simulink model "LABVALVSIMU2019a"  (R2019b)
settings: Solver=VariableStepAuto  StartTime=0.0  StopTime=50  RelTol=1e-3  EnableMultiTasking=on
libraries: simulink x1
settings Model: Creator=mateog  LastModifiedBy=gesro
settings DataIOCC: ReturnWorkspaceOutputs=off
settings OptimizationCC: LifeSpan=inf
settings DebuggingCC: SFUnexpectedBacktrackingDiag=warning  SFNoUnconditionalDefaultTransitionDiag=warning  ArithmeticOperatorsInVariantConditions=warning
settings SFSimCC: SimUseLocalCustomCode=off  CustomCodeUndefinedFunction=UseInterfaceOnly
settings RTWCC: RTWUseLocalCustomCode=off
settings CodeAppCC: StateflowObjectComments=on
settings GRTTargetCC: TargetLangStandard=C89/C90 (ANSI)
settings ConfigComp: CovMetricSettings=dw  CovHtmlReporting=on  CovSaveCumulativeToWorkspaceVar=on  CovSaveSingleToWorkspaceVar=on  CovExternalEMLEnable=off

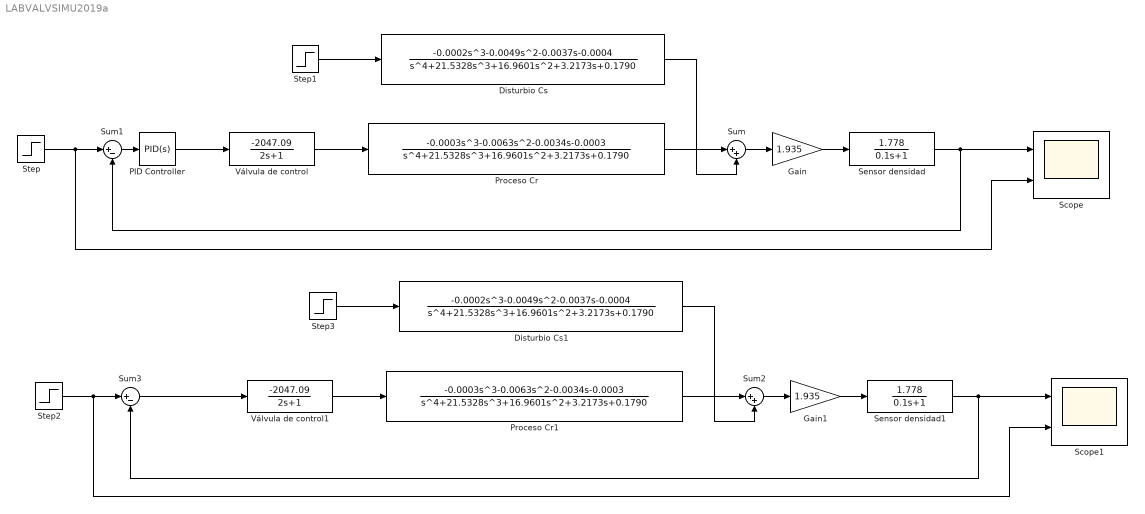
== system LABVALVSIMU2019a ==
  Disturbio Cs : TransferFcn  Numerator=[-0.0002 -0.0049 -0.0037 -0.0004]  Denominator=[1 21.5328 16.9601 3.2173 0.1790]
  Disturbio Cs1 : TransferFcn  Numerator=[-0.0002 -0.0049 -0.0037 -0.0004]  Denominator=[1 21.5328 16.9601 3.2173 0.1790]
  Gain : Gain  Gain=1.935
  Gain1 : Gain  Gain=1.935
  PID Controller : simulink/Continuous/PID Controller  Controller=PID  Form=Ideal  TimeDomain=Continuous-time  SampleTime=-1  IntegratorMethod=Forward Euler  FilterMethod=Forward Euler  ControllerParametersSource=internal  P=0.955917062218505  I=0.151469512178024  D=1.64233942236467  UseFilter=on  N=100  TunerSelectOption=Transfer Function Based (PID Tuner App)  InitialConditionSource=internal  InitialConditionForIntegrator=0  InitialConditionForFilter=0  DifferentiatorICPrevScaledInput=0  ExternalReset=none  TrackingMode=off  Kt=1  LimitOutput=off  UpperSaturationLimit=inf  LowerSaturationLimit=-inf  LinearizeAsGain=on  AntiWindupMode=none  Kb=1  POutMin=[]  POutMax=[]  IOutMin=[]  IOutMax=[]  DOutMin=[]  DOutMax=[]  NOutMin=[]  NOutMax=[]  SumOutMin=[]  SumOutMax=[]  SaturationOutMin=[]  SaturationOutMax=[]  PParamMin=[]  PParamMax=[]  IParamMin=[]  IParamMax=[]  DParamMin=[]  DParamMax=[]  NParamMin=[]  NParamMax=[]  KbParamMin=[]  KbParamMax=[]  KtParamMin=[]  KtParamMax=[]  KbOutMin=[]  KbOutMax=[]  KtOutMin=[]  KtOutMax=[]  IntegratorOutMin=[]  IntegratorOutMax=[]  FilterOutMin=[]  FilterOutMax=[]  SumI1OutMin=[]  SumI1OutMax=[]  SumI2OutMin=[]  SumI2OutMax=[]  SumI3OutMin=[]  SumI3OutMax=[]  SumI4OutMin=[]  SumI4OutMax=[]  SumDOutMin=[]  SumDOutMax=[]  DifferentiatorOutMin=[]  DifferentiatorOutMax=[]  FilterDiffOutCoefMin=[]  FilterDiffOutCoefMax=[]  ReciprocalOutMin=[]  ReciprocalOutMax=[]  SumDenOutMin=[]  SumDenOutMax=[]  SumNumOutMin=[]  SumNumOutMax=[]  DivideOutMin=[]  DivideOutMax=[]  IntegratorContinuousStateAttributes=''  IntegratorStateMustResolveToSignalObject=off  IntegratorRTWStateStorageClass=Auto  FilterContinuousStateAttributes=''  FilterStateMustResolveToSignalObject=off  FilterRTWStateStorageClass=Auto  ParallelPVariant=Passthrough  IdealPVariant=InternalParameters  IVariant=InternalParameters  DVariant=InternalParameters  IntegratorVariant=Continuous  SatVariant=Disabled  AWVariant=Passthrough  PCopyVariant=Disabled  TRVariant=Disabled  FdbkBlocksVariant=Forward  IdealPFdbkVariant=Disabled  SatFdbkVariant=Disabled  DerivativeFilterVariant=ContFilter  NVariant=InternalParameters  NCopyVariant=Disabled  FilterICVariant=InternalICsFilter  IntegratorICVariant=InternalICs  ExternalResetVariant=Disabled  TRSumVariant=Passthrough  SumFdbkVariant=Disabled  SumVariant=Sum_PID
  Proceso Cr : TransferFcn  Numerator=[-0.0003 -0.0063 -0.0034 -0.0003]  Denominator=[1 21.5328 16.9601 3.2173 0.1790]
  Proceso Cr1 : TransferFcn  Numerator=[-0.0003 -0.0063 -0.0034 -0.0003]  Denominator=[1 21.5328 16.9601 3.2173 0.1790]
  Scope : Scope  NumInputPorts=2
  Scope1 : Scope  NumInputPorts=2
  Sensor densidad : TransferFcn  Numerator=[1.778]  Denominator=[0.1 1]
  Sensor densidad1 : TransferFcn  Numerator=[1.778]  Denominator=[0.1 1]
  Step{,1..3} (4 alike) : Step  SampleTime=0
  Sum : Sum  Inputs=|++
  Sum1 : Sum  Inputs=|+-
  Sum2 : Sum  Inputs=|++
  Sum3 : Sum  Inputs=|+-
  Válvula de control : TransferFcn  Numerator=[-2047.09]  Denominator=[2 1]
  Válvula de control1 : TransferFcn  Numerator=[-2047.09]  Denominator=[2 1]
  wires:
  Sum/1 -> Gain/1
  Válvula de control/1 -> Proceso Cr/1
  Step1/1 -> Disturbio Cs/1
  Proceso Cr/1 -> Sum/1
  PID Controller/1 -> Válvula de control/1
  Sum1/1 -> PID Controller/1
  Step/1 -> Scope/2, Sum1/1
  Disturbio Cs/1 -> Sum/2
  Sensor densidad/1 -> Sum1/2, Scope/1
  Gain/1 -> Sensor densidad/1
  Válvula de control1/1 -> Proceso Cr1/1
  Gain1/1 -> Sensor densidad1/1
  Sum2/1 -> Gain1/1
  Sum3/1 -> Válvula de control1/1
  Step3/1 -> Disturbio Cs1/1
  Sensor densidad1/1 -> Sum3/2, Scope1/1
  Proceso Cr1/1 -> Sum2/1
  Disturbio Cs1/1 -> Sum2/2
  Step2/1 -> Scope1/2, Sum3/1
